simulink model "wec_qlearning"  (R2017b)
settings: Solver=VariableStepAuto  StartTime=0.0  StopTime=100.0  RelTol=1e-3
values from neighbouring files (symbols this model uses):
  B = zeros(vz,hz)    [ACTOR_CRITIC & SARSA.m]    (also in InputDataExtraction.m = 0.01; TDlearningExampleEforPosting.m)
  K = K_stiff*133333    (= 199999.5)    [InputDataExtraction.m]
  m = min(Out,[],2)    [ContinousControl.m]    (also in RL.m; RealTime_modif22.m)
undefined symbols (not defined in the file or in its folder): A, dzb_0, wp, zb_0
settings Model: Creator=brekken  LastModifiedBy=ghleila
settings CodeAppCC: StateflowObjectComments=on

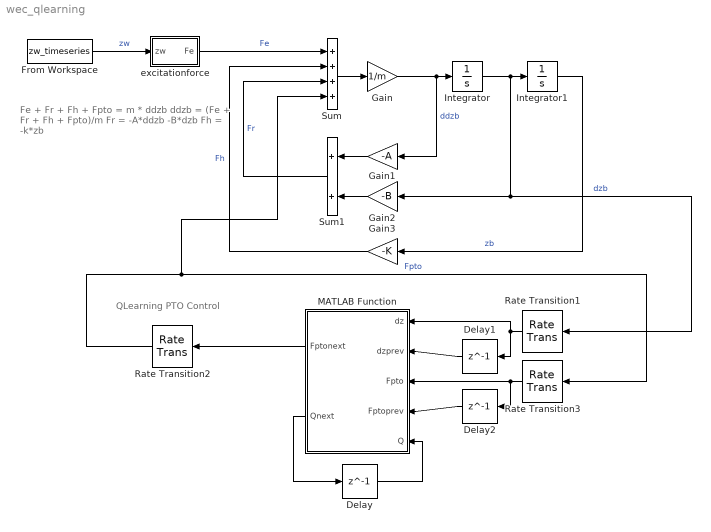
== system wec_qlearning ==
  note: QLearning PTO Control
  note: Fe + Fr + Fh + Fpto = m * ddzb
      | ddzb = (Fe + Fr + Fh + Fpto)/m
      |
      | Fr = -A*ddzb -B*dzb
      |
      | Fh = -k*zb
  Delay : Delay  DelayLength=1
  Delay1 : Delay  DelayLength=1
  Delay2 : Delay  DelayLength=1
  From Workspace : FromWorkspace  VariableName=zw_timeseries  SampleTime=0
  Gain : Gain  Gain=1/m
  Gain1 : Gain  Gain=-A
  Gain2 : Gain  Gain=-B
  Gain3 : Gain  Gain=-K
  Integrator : Integrator  InitialCondition=dzb_0
  Integrator1 : Integrator  InitialCondition=zb_0
  MATLAB Function : MATLAB Function  TreatAsAtomicUnit=on
  Rate Transition1 : RateTransition  Deterministic=off  OutPortSampleTime=QSampleTime
  Rate Transition2 : RateTransition  Deterministic=off  OutPortSampleTime=0
  Rate Transition3 : RateTransition  Deterministic=off  OutPortSampleTime=QSampleTime
  Sum : Sum  Inputs=++++
  Sum1 : Sum
  excitationforce : Subsystem
  wires:
  Gain/1 -> Gain1/1, Integrator/1  "ddzb"
  Integrator/1 -> Rate Transition1/1, Gain2/1, Integrator1/1  "dzb"
  Integrator1/1 -> Gain3/1  "zb"
  Sum/1 -> Gain/1
  Sum1/1 -> Sum/3  "Fr"
  Gain3/1 -> Sum/2  "Fh"
  Rate Transition2/1 -> Sum/4, Rate Transition3/1  "Fpto"
  Gain1/1 -> Sum1/1
  Gain2/1 -> Sum1/2
  From Workspace/1 -> excitationforce/1(zw)  "zw"
  excitationforce/1(Fe) -> Sum/1  "Fe"
  Rate Transition1/1 -> Delay1/1, MATLAB Function/1(dz)
  MATLAB Function/2(Qnext) -> Delay/1
  Delay1/1 -> MATLAB Function/2(dzprev)
  Rate Transition3/1 -> Delay2/1, MATLAB Function/3(Fpto)
  Delay2/1 -> MATLAB Function/4(Fptoprev)
  Delay/1 -> MATLAB Function/5(Q)
  MATLAB Function/1(Fptonext) -> Rate Transition2/1

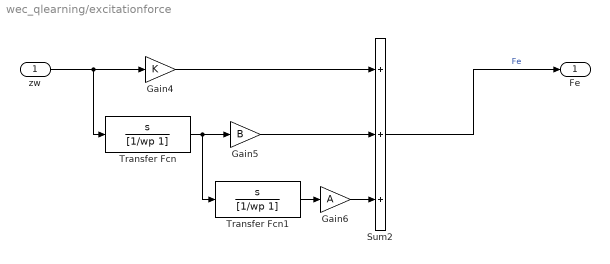
== system wec_qlearning/excitationforce ==
  zw : Inport
  Gain4 : Gain  Gain=K
  Gain5 : Gain  Gain=B
  Gain6 : Gain  Gain=A
  Sum2 : Sum  Inputs=+++
  Transfer Fcn : TransferFcn  Numerator=[1 0]  Denominator=[1/wp 1]
  Transfer Fcn1 : TransferFcn  Numerator=[1 0]  Denominator=[1/wp 1]
  Fe : Outport
  wires:
  Transfer Fcn/1 -> Transfer Fcn1/1, Gain5/1
  Gain5/1 -> Sum2/2
  Gain6/1 -> Sum2/3
  Sum2/1 -> Fe/1  "Fe"
  zw/1 -> Transfer Fcn/1, Gain4/1
  Transfer Fcn1/1 -> Gain6/1
  Gain4/1 -> Sum2/1

== matlab function wec_qlearning/MATLAB Function ==
  data: Fptonext output; dz input; dzprev input; Fpto input; Fptoprev input; Q input; Qnext output
function [Fptonext, Qnext] = fcn(dz,dzprev,Fpto,Fptoprev,Q)

% From https://web.stanford.edu/group/pdplab/pdphandbook/handbookch10.html
% Q(s,a) = Q(s,a)*(1-learningRate) 
%          + learningRate*(r1 + discountFactor*Q(s1,a1))
%
% Q is value of being in a state and taking that action in that state
% Reward is reward of being in that state AND taking that action 
% (Not the reward of being in a state)

learningRate = 0.5;
discountFactor = 0.5;
